simulink model "Q4_Sensor_Unpack"  (R2018b)
settings: Solver=VariableStepAuto  StartTime=0.0  StopTime=10.0  RelTol=1e-3
(part 2 of 2)

== matlab function Q4_Sensor_Unpack/message_unpack ==
  data: CAFDva_y_F_RadarData151 input; CAFDva_y_F_RadarData152 input; CAFDva_y_F_RadarData153 input; CAFDva_y_F_RadarData154 input; CAFDva_y_F_RadarData155 input; CAFDva_y_F_RadarData156 input; CAFDva_y_F_RadarData157 input; CAFDva_y_F_RadarData158 input; CAFDva_y_F_RadarData159 input; CAFDva_y_F_RadarData15A input; CAFDva_y_F_RadarData15B input; CAFDva_y_F_RadarData15C input; CAFDva_y_F_RadarData15D input; CAFDva_y_F_RadarData15E input; CAFDva_y_F_RadarData15F input; CAFDva_y_F_RadarData160 input; CAFDva_y_F_RadarData161 input; CAFDva_y_F_RadarData162 input; CAFDva_y_F_RadarData163 input; CAFDva_y_F_RadarData164 input; CAFDva_y_F_RadarData165 input; CAFDva_y_F_RadarData166 input; CAFDva_y_F_RadarData167 input; CAFDva_y_F_RadarData168 input; CAFDva_y_F_RadarData169 input; CAFDva_y_F_CameraData600 input; CAFDva_y_F_CameraData424 input; CAFDva_y_F_CameraData425 input; CAFDva_y_F_CameraData450 input; CAFDva_y_F_CameraData459 input; CAFDva_y_F_CameraData45A input; CAFDva_y_F_CameraData45B input; CAFDva_y_F_CameraData45C input; CAFDva_y_F_CameraData45D input; CAFDva_y_F_CameraData45E input; CAFDva_y_F_CameraData45F input; CAFDva_y_F_CameraData420 input; CAFDva_y_F_CameraData421 input; CAFDva_y_F_CameraData422 input; CAFDva_y_F_CameraData451 input; CAFDva_y_F_CameraData423 input; CAFDva_y_F_CameraData452 input; CAFDva_y_F_CameraData453 input; CAFDva_y_F_CameraData454 input; CAFDva_y_F_CameraData455 input; CAFDva_y_F_CameraData456 input; CAFDva_y_F_CameraData457 input; CAFDva_y_F_CameraData458 input; CAFDva_y_F_CameraData426 input; Radar_Timestamp output; Radar_status output; Radar_num output; Radar_P_long output; Radar_P_long_std output; Radar_P_latd output; Radar_P_latd_std output; Radar_P_Dis_cov output; Radar_Relative_V_long output; Radar_Relative_V_lat output; Radar_Relative_Acc_lat output; Radar_Relative_Acc_long output; Radar_Abs_V_long output; Radar_Abs_V_long_std output; Radar_Abs_V_long_acc output; Radar_Abs_V_long_acc_std output; Radar_Abs_V_lat output; Radar_Abs_V_lat_std output; Radar_Abs_V_lat_acc output; Radar_Abs_V_lat_acc_std output; Radar_Abs_V_cov output; Radar_Abs_V_acc_cov output; Radar_Class_type output; Radar_Class_prob output; Radar_Obj_length output; Radar_Obj_length_std output; Radar_Obj_width output; Radar_Obj_width_std output; Radar_Obj_height output; Radar_Obj_height_std output; Radar_Obj_id output; Radar_Obj_age output; Radar_Obj_referpoint output; Radar_Obj_Yaw output; Radar_Obj_Yaw_std output; Radar_Obj_Movementstatus output; Radar_Obj_Measurestatus output; Radar_Braking_allowed output; Radar_CrossSection output; Radar_Exist_prob output; IFC_obj_timestamp output; IFC_State output; IFC_ObjHdr_ObjCount output; IFC_VD_CIPV_ID output; FS_Out_Of_Calib output; FS_Rain output; FS_Fog output; FS_Splashes_0 output; FS_Sun_Ray_0 output; FS_Low_Sun_0 output; FS_Blur_Image_0 output; FS_Partial_Blockage_0 output; FS_Full_Blockage_0 output; FS_Frozen_Windshield_0 output; FS_Out_Of_Focus_0 output; IFC_obj_TTIPC_StdDev output; IFC_obj_abs_Ax output; IFC_obj_abs_Ay output; IFC_obj_Rel_Vx output; IFC_obj_Rel_Vy output; IFC_obj_Dx output; IFC_obj_Dy output; IFC_obj_abs_AxStdDev output; IFC_obj_abs_AyStdDev output; IFC_obj_Rel_VxStdDev output; IFC_obj_Rel_VyStdDev output; IFC_obj_DxStdDev output; IFC_obj_DyStdDev output; IFC_obj_Rel_VxValid output; IFC_obj_Rel_VyValid output; IFC_obj_Rel_VxStdDevValid output; IFC_obj_Rel_VyStdDevValid output; IFC_obj_ExistProb output; IFC_obj_TypeProb output; IFC_obj_Width output; IFC_obj_Height output; IFC_obj_LengthStdDev output; IFC_obj_WidthStdDev output; IFC_obj_HeightStdDev output; IFC_obj_PhiLeft output; IFC_obj_PhiRight output; IFC_obj_angle_3D output; IFC_obj_PhiLeftStdDev output; IFC_obj_PhiRightStdDev output; IFC_obj_angle_3DStdDev output; IFC_obj_angle_rate output; IFC_obj_angle_rate_StdDev output; IFC_obj_PhiBottom output; IFC_obj_PhiBottomStdDev output; IFC_obj_Measured output; IFC_obj_Heading output; IFC_obj_HeadingStdDev output; IFC_obj_HeadOrientation output; IFC_obj_Type output; IFC_obj_ID output; IFC_obj_TTIPC output; IFC_obj_DirIndicator output; IFC_obj_BrakeLight output; IFC_Line01_LineID output; IFC_Line01_ExistProb output; IFC_Line01_DxStart output; IFC_Line01_ColorClass output; IFC_Line01_DxEnd output; IFC_Line01_HeadingAngle output; IFC_Line01_Dy output; IFC_Line01_CurvChange output; IFC_Line01_Curv output; IFC_Line01_MeasureType output; IFC_Line01_LineWidth output; IFC_Line01_Type output; IFC_Line01_TypeConf output; IFC_Line02_LineID output; IFC_Line02_ExistProb output; IFC_Line02_DxStart output; IFC_Line02_ColorClass output; IFC_Line02_DxEnd output; IFC_Line02_HeadingAngle output; IFC_Line02_Dy output; IFC_Line02_CurvChange output; IFC_Line02_Curv output; IFC_Line02_MeasureType output; IFC_Line02_LineWidth output; IFC_Line02_Type output; IFC_Line02_TypeConf output; IFC_Line03_LineID output; IFC_Line03_ExistProb output; IFC_Line03_DxStart output; IFC_Line03_ColorClass output; IFC_Line03_DxEnd output; IFC_Line03_HeadingAngle output; IFC_Line03_Dy output; IFC_Line03_CurvChange output; IFC_Line03_Curv output; IFC_Line03_MeasureType output; IFC_Line03_LineWidth output; IFC_Line03_Type output; IFC_Line03_TypeConf output; IFC_Line04_LineID output; IFC_Line04_ExistProb output; IFC_Line04_DxStart output; IFC_Line04_ColorClass output; IFC_Line04_DxEnd output; IFC_Line04_HeadingAngle output; IFC_Line04_Dy output; IFC_Line04_CurvChange output; IFC_Line04_Curv output; IFC_Line04_MeasureType output; IFC_Line04_LineWidth output; IFC_Line04_Type output; IFC_Line04_TypeConf output; IFC_Roadedge01_LineID output; IFC_Roadedge01_ExistProb output; IFC_Roadedge01_DxStart output; IFC_Roadedge01_DxEnd output; IFC_Roadedge01_HeadingAngle output; IFC_Roadedge01_Dy output; IFC_Roadedge01_Curv output; IFC_Roadedge01_CurvChange output; IFC_Roadedge01_MeasureType output; IFC_Roadedge01_Type output; IFC_Roadedge02_LineID output; IFC_Roadedge02_ExistProb output; IFC_Roadedge02_DxStart output; IFC_Roadedge02_DxEnd output; IFC_Roadedge02_HeadingAngle output; IFC_Roadedge02_Dy output; IFC_Roadedge02_Curv output; IFC_Roadedge02_CurvChange output; IFC_Roadedge02_MeasureType output; IFC_Roadedge02_Type output; CAFDva_y_F_CameraData47E input
%% function for unpack and repack of canfd log data by liuyij 20210224
function [Radar_Timestamp,Radar_status,Radar_num,Radar_P_long,Radar_P_long_std,Radar_P_latd,Radar_P_latd_std,Radar_P_Dis_cov,...
    Radar_Relative_V_long,Radar_Relative_V_lat,Radar_Relative_Acc_lat,Radar_Relative_Acc_long,Radar_Abs_V_long,...
    Radar_Abs_V_long_std,Radar_Abs_V_long_acc,Radar_Abs_V_long_acc_std,Radar_Abs_V_lat,Radar_Abs_V_lat_std,Radar_Abs_V_lat_acc,...
    Radar_Abs_V_lat_acc_std,Radar_Abs_V_cov,Radar_Abs_V_acc_cov,Radar_Class_type,Radar_Class_prob,Radar_Obj_length,Radar_Obj_length_std,...
    Radar_Obj_width,Radar_Obj_width_std,Radar_Obj_height,Radar_Obj_height_std,Radar_Obj_id,Radar_Obj_age,Radar_Obj_referpoint,Radar_Obj_Yaw,...
    Radar_Obj_Yaw_std,Radar_Obj_Movementstatus,Radar_Obj_Measurestatus,Radar_Braking_allowed,Radar_CrossSection,Radar_Exist_prob,...
    IFC_obj_timestamp,IFC_State,IFC_ObjHdr_ObjCount,IFC_VD_CIPV_ID,...
    FS_Out_Of_Calib,FS_Rain,FS_Fog,FS_Splashes_0,FS_Sun_Ray_0,FS_Low_Sun_0,FS_Blur_Image_0,FS_Partial_Blockage_0,FS_Full_Blockage_0,FS_Frozen_Windshield_0,FS_Out_Of_Focus_0,...
    IFC_obj_TTIPC_StdDev,IFC_obj_abs_Ax,IFC_obj_abs_Ay,IFC_obj_Rel_Vx,IFC_obj_Rel_Vy,IFC_obj_Dx,IFC_obj_Dy,IFC_obj_abs_AxStdDev,IFC_obj_abs_AyStdDev,...
    IFC_obj_Rel_VxStdDev,IFC_obj_Rel_VyStdDev,IFC_obj_DxStdDev,IFC_obj_DyStdDev,IFC_obj_Rel_VxValid,IFC_obj_Rel_VyValid,IFC_obj_Rel_VxStdDevValid,...
    IFC_obj_Rel_VyStdDevValid,IFC_obj_ExistProb,IFC_obj_TypeProb,IFC_obj_Width,IFC_obj_Height,IFC_obj_LengthStdDev,IFC_obj_WidthStdDev,IFC_obj_HeightStdDev,...
    IFC_obj_PhiLeft,IFC_obj_PhiRight,IFC_obj_angle_3D,IFC_obj_PhiLeftStdDev,IFC_obj_PhiRightStdDev,IFC_obj_angle_3DStdDev,IFC_obj_angle_rate,...
    IFC_obj_angle_rate_StdDev,IFC_obj_PhiBottom,IFC_obj_PhiBottomStdDev,IFC_obj_Measured,IFC_obj_Heading,IFC_obj_HeadingStdDev,IFC_obj_HeadOrientation,...
    IFC_obj_Type,IFC_obj_ID,IFC_obj_TTIPC,IFC_obj_DirIndicator,IFC_obj_BrakeLight,...
    IFC_Line01_LineID,IFC_Line01_ExistProb,IFC_Line01_DxStart,IFC_Line01_ColorClass,IFC_Line01_DxEnd,IFC_Line01_HeadingAngle,IFC_Line01_Dy,...
    IFC_Line01_CurvChange,IFC_Line01_Curv,IFC_Line01_MeasureType,IFC_Line01_LineWidth,IFC_Line01_Type,IFC_Line01_TypeConf,...
    IFC_Line02_LineID,IFC_Line02_ExistProb,IFC_Line02_DxStart,IFC_Line02_ColorClass,IFC_Line02_DxEnd,IFC_Line02_HeadingAngle,IFC_Line02_Dy,...
    IFC_Line02_CurvChange,IFC_Line02_Curv,IFC_Line02_MeasureType,IFC_Line02_LineWidth,IFC_Line02_Type,IFC_Line02_TypeConf,...
    IFC_Line03_LineID,IFC_Line03_ExistProb,IFC_Line03_DxStart,IFC_Line03_ColorClass,IFC_Line03_DxEnd,IFC_Line03_HeadingAngle,IFC_Line03_Dy,...
    IFC_Line03_CurvChange,IFC_Line03_Curv,IFC_Line03_MeasureType,IFC_Line03_LineWidth,IFC_Line03_Type,IFC_Line03_TypeConf,...
    IFC_Line04_LineID,IFC_Line04_ExistProb,IFC_Line04_DxStart,IFC_Line04_ColorClass,IFC_Line04_DxEnd,IFC_Line04_HeadingAngle,IFC_Line04_Dy,...
    IFC_Line04_CurvChange,IFC_Line04_Curv,IFC_Line04_MeasureType,IFC_Line04_LineWidth,IFC_Line04_Type,IFC_Line04_TypeConf,...
    IFC_Roadedge01_LineID,IFC_Roadedge01_ExistProb,IFC_Roadedge01_DxStart,IFC_Roadedge01_DxEnd,IFC_Roadedge01_HeadingAngle,...
    IFC_Roadedge01_Dy,IFC_Roadedge01_Curv,IFC_Roadedge01_CurvChange,IFC_Roadedge01_MeasureType,IFC_Roadedge01_Type,...
    IFC_Roadedge02_LineID,IFC_Roadedge02_ExistProb,IFC_Roadedge02_DxStart,IFC_Roadedge02_DxEnd,IFC_Roadedge02_HeadingAngle,...
    IFC_Roadedge02_Dy,IFC_Roadedge02_Curv,IFC_Roadedge02_CurvChange,IFC_Roadedge02_MeasureType,IFC_Roadedge02_Type]...
    = sensor_unpack(CAFDva_y_F_RadarData151,CAFDva_y_F_RadarData152,CAFDva_y_F_RadarData153,CAFDva_y_F_RadarData154,...
    CAFDva_y_F_RadarData155,CAFDva_y_F_RadarData156,CAFDva_y_F_RadarData157,CAFDva_y_F_RadarData158,CAFDva_y_F_RadarData159,...
    CAFDva_y_F_RadarData15A,CAFDva_y_F_RadarData15B,CAFDva_y_F_RadarData15C,CAFDva_y_F_RadarData15D,CAFDva_y_F_RadarData15E,CAFDva_y_F_RadarData15F,...
    CAFDva_y_F_RadarData160,CAFDva_y_F_RadarData161,CAFDva_y_F_RadarData162,CAFDva_y_F_RadarData163,CAFDva_y_F_RadarData164,...
    CAFDva_y_F_RadarData165,CAFDva_y_F_RadarData166,CAFDva_y_F_RadarData167,CAFDva_y_F_RadarData168,CAFDva_y_F_RadarData169,...
    CAFDva_y_F_CameraData600,CAFDva_y_F_CameraData424,CAFDva_y_F_CameraData425,CAFDva_y_F_CameraData450,CAFDva_y_F_CameraData459,...
    CAFDva_y_F_CameraData45A,CAFDva_y_F_CameraData45B,CAFDva_y_F_CameraData45C,CAFDva_y_F_CameraData45D,CAFDva_y_F_CameraData45E,...
    CAFDva_y_F_CameraData45F,CAFDva_y_F_CameraData420,CAFDva_y_F_CameraData421,CAFDva_y_F_CameraData422,CAFDva_y_F_CameraData451,...
    CAFDva_y_F_CameraData423,CAFDva_y_F_CameraData452,CAFDva_y_F_CameraData453,CAFDva_y_F_CameraData454,CAFDva_y_F_CameraData455,...
    CAFDva_y_F_CameraData456,CAFDva_y_F_CameraData457,CAFDva_y_F_CameraData458,CAFDva_y_F_CameraData426,CAFDva_y_F_CameraData47E)

RADAR_MAX = uint8(24);
CAM_MAX = uint8(20);

%% output data initial 
% radar output
Radar_Timestamp = zeros(RADAR_MAX,1,'uint16');
Radar_status = uint8(0);
Radar_num = uint8(0);
Radar_P_long = zeros(RADAR_MAX,1,'single');
Radar_P_long_std= zeros(RADAR_MAX,1,'single');
Radar_P_latd= zeros(RADAR_MAX,1,'single');
Radar_P_latd_std= zeros(RADAR_MAX,1,'single');
Radar_P_Dis_cov= zeros(RADAR_MAX,1,'single');
Radar_Relative_V_long= zeros(RADAR_MAX,1,'single');
Radar_Relative_V_lat= zeros(RADAR_MAX,1,'single');
Radar_Relative_Acc_lat= zeros(RADAR_MAX,1,'single');
Radar_Relative_Acc_long= zeros(RADAR_MAX,1,'single');
Radar_Abs_V_long= zeros(RADAR_MAX,1,'single');
Radar_Abs_V_long_std= zeros(RADAR_MAX,1,'single');
Radar_Abs_V_long_acc= zeros(RADAR_MAX,1,'single');
Radar_Abs_V_long_acc_std= zeros(RADAR_MAX,1,'single');
Radar_Abs_V_lat= zeros(RADAR_MAX,1,'single');
Radar_Abs_V_lat_std= zeros(RADAR_MAX,1,'single');
Radar_Abs_V_lat_acc= zeros(RADAR_MAX,1,'single');
Radar_Abs_V_lat_acc_std= zeros(RADAR_MAX,1,'single');
Radar_Abs_V_cov= zeros(RADAR_MAX,1,'single');
Radar_Abs_V_acc_cov = zeros(RADAR_MAX,1,'single');
Radar_Class_type= zeros(RADAR_MAX,1,'uint8');
Radar_Class_prob= zeros(RADAR_MAX,1,'uint8');
Radar_Obj_length = zeros(RADAR_MAX,1,'single');
Radar_Obj_length_std = zeros(RADAR_MAX,1,'single');
Radar_Obj_width = zeros(RADAR_MAX,1,'single');
Radar_Obj_width_std = zeros(RADAR_MAX,1,'single');
Radar_Obj_height = zeros(RADAR_MAX,1,'single');
Radar_Obj_height_std = zeros(RADAR_MAX,1,'single');
Radar_Obj_id = zeros(RADAR_MAX,1,'uint8');
Radar_Obj_age = zeros(RADAR_MAX,1,'single');
Radar_Obj_referpoint = zeros(RADAR_MAX,1,'uint8');
Radar_Obj_Yaw = zeros(RADAR_MAX,1,'single');
Radar_Obj_Yaw_std = zeros(RADAR_MAX,1,'single');
Radar_Obj_Movementstatus = zeros(RADAR_MAX,1,'uint8');
Radar_Obj_Measurestatus = zeros(RADAR_MAX,1,'uint8');
Radar_Braking_allowed = zeros(RADAR_MAX,1,'uint8');
Radar_CrossSection = zeros(RADAR_MAX,1,'single');
Radar_Exist_prob = zeros(RADAR_MAX,1,'uint8');

% cam output
IFC_State = zeros(1,1,'uint8');
IFC_ObjHdr_ObjCount = zeros(1,1,'uint8');
IFC_VD_CIPV_ID = zeros(1,1,'uint8');

FS_Out_Of_Calib = zeros(1,1,'uint8');
FS_Rain = zeros(1,1,'uint8');
FS_Fog = zeros(1,1,'uint8');
FS_Splashes_0 = zeros(1,1,'uint8');
FS_Sun_Ray_0 = zeros(1,1,'uint8');
FS_Low_Sun_0 = zeros(1,1,'uint8');
FS_Blur_Image_0 = zeros(1,1,'uint8');
FS_Partial_Blockage_0 = zeros(1,1,'uint8');
FS_Full_Blockage_0 = zeros(1,1,'uint8');
FS_Frozen_Windshield_0 = zeros(1,1,'uint8');
FS_Out_Of_Focus_0 = zeros(1,1,'uint8');

IFC_obj_TTIPC_StdDev = zeros(CAM_MAX,1,'single');
IFC_obj_abs_Ax = zeros(CAM_MAX,1,'single');
IFC_obj_abs_Ay = zeros(CAM_MAX,1,'single');
IFC_obj_Rel_Vx = zeros(CAM_MAX,1,'single');
IFC_obj_Rel_Vy = zeros(CAM_MAX,1,'single');
IFC_obj_Dx = zeros(CAM_MAX,1,'single');
IFC_obj_Dy = zeros(CAM_MAX,1,'single');
IFC_obj_abs_AxStdDev = zeros(CAM_MAX,1,'single');
IFC_obj_abs_AyStdDev = zeros(CAM_MAX,1,'single');
IFC_obj_Rel_VxStdDev = zeros(CAM_MAX,1,'single');
IFC_obj_Rel_VyStdDev = zeros(CAM_MAX,1,'single');
IFC_obj_DxStdDev = zeros(CAM_MAX,1,'single');
IFC_obj_DyStdDev = zeros(CAM_MAX,1,'single');
IFC_obj_Rel_VxValid = zeros(CAM_MAX,1,'uint8');
IFC_obj_Rel_VyValid = zeros(CAM_MAX,1,'uint8');
IFC_obj_Rel_VxStdDevValid = zeros(CAM_MAX,1,'uint8');
IFC_obj_Rel_VyStdDevValid = zeros(CAM_MAX,1,'uint8');
IFC_obj_ExistProb = zeros(CAM_MAX,1,'single');
IFC_obj_TypeProb = zeros(CAM_MAX,1,'single');
IFC_obj_Width = zeros(CAM_MAX,1,'single');
IFC_obj_Height = zeros(CAM_MAX,1,'single');
IFC_obj_LengthStdDev = zeros(CAM_MAX,1,'single');
IFC_obj_WidthStdDev = zeros(CAM_MAX,1,'single');
IFC_obj_HeightStdDev = zeros(CAM_MAX,1,'single');
IFC_obj_PhiLeft = zeros(CAM_MAX,1,'single');
IFC_obj_PhiRight = zeros(CAM_MAX,1,'single');
IFC_obj_angle_3D = zeros(CAM_MAX,1,'single');
IFC_obj_PhiLeftStdDev = zeros(CAM_MAX,1,'single');
IFC_obj_PhiRightStdDev = zeros(CAM_MAX,1,'single');
IFC_obj_angle_3DStdDev = zeros(CAM_MAX,1,'single');
IFC_obj_angle_rate = zeros(CAM_MAX,1,'single');
IFC_obj_angle_rate_StdDev = zeros(CAM_MAX,1,'single');
IFC_obj_PhiBottom = zeros(CAM_MAX,1,'single');
IFC_obj_PhiBottomStdDev = zeros(CAM_MAX,1,'single');
IFC_obj_Measured = zeros(CAM_MAX,1,'uint8');
IFC_obj_Heading = zeros(CAM_MAX,1,'single');
IFC_obj_HeadingStdDev = zeros(CAM_MAX,1,'single');
IFC_obj_HeadOrientation = zeros(CAM_MAX,1,'uint8');
IFC_obj_Type = zeros(CAM_MAX,1,'uint8');
IFC_obj_ID = zeros(CAM_MAX,1,'uint8');
IFC_obj_TTIPC = zeros(CAM_MAX,1,'single');
IFC_obj_DirIndicator = zeros(CAM_MAX,1,'uint8');
IFC_obj_BrakeLight = zeros(CAM_MAX,1,'uint8');

IFC_obj_timestamp = zeros(CAM_MAX,1,'uint16');

IFC_Line01_LineID = zeros(1,1,'uint8');
IFC_Line01_ExistProb = zeros(1,1,'single');
IFC_Line01_DxStart = zeros(1,1,'single');
IFC_Line01_ColorClass = zeros(1,1,'uint8');
IFC_Line01_DxEnd = zeros(1,1,'single');
IFC_Line01_HeadingAngle = zeros(1,1,'single');
IFC_Line01_Dy = zeros(1,1,'single');
IFC_Line01_CurvChange = zeros(1,1,'single');
IFC_Line01_Curv = zeros(1,1,'single');
IFC_Line01_MeasureType = zeros(1,1,'uint8');
IFC_Line01_LineWidth = zeros(1,1,'single');
IFC_Line01_Type = zeros(1,1,'uint8');
IFC_Line01_TypeConf = zeros(1,1,'single');
IFC_Line02_LineID = zeros(1,1,'uint8');
IFC_Line02_ExistProb = zeros(1,1,'single');
IFC_Line02_DxStart = zeros(1,1,'single');
IFC_Line02_ColorClass = zeros(1,1,'uint8');
IFC_Line02_DxEnd = zeros(1,1,'single');
IFC_Line02_HeadingAngle = zeros(1,1,'single');
IFC_Line02_Dy = zeros(1,1,'single');
IFC_Line02_CurvChange = zeros(1,1,'single');
IFC_Line02_Curv = zeros(1,1,'single');
IFC_Line02_MeasureType = zeros(1,1,'uint8');
IFC_Line02_LineWidth = zeros(1,1,'single');
IFC_Line02_Type = zeros(1,1,'uint8');
IFC_Line02_TypeConf = zeros(1,1,'single');

IFC_Line03_LineID = zeros(1,1,'uint8');
IFC_Line03_ExistProb = zeros(1,1,'single');
IFC_Line03_DxStart = zeros(1,1,'single');
IFC_Line03_ColorClass = zeros(1,1,'uint8');
IFC_Line03_DxEnd = zeros(1,1,'single');
IFC_Line03_HeadingAngle = zeros(1,1,'single');
IFC_Line03_Dy = zeros(1,1,'single');
IFC_Line03_CurvChange = zeros(1,1,'single');
IFC_Line03_Curv = zeros(1,1,'single');
IFC_Line03_MeasureType = zeros(1,1,'uint8');
IFC_Line03_LineWidth = zeros(1,1,'single');
IFC_Line03_Type = zeros(1,1,'uint8');
IFC_Line03_TypeConf = zeros(1,1,'single');
IFC_Line04_LineID = zeros(1,1,'uint8');
IFC_Line04_ExistProb = zeros(1,1,'single');
IFC_Line04_DxStart = zeros(1,1,'single');
IFC_Line04_ColorClass = zeros(1,1,'uint8');
IFC_Line04_DxEnd = zeros(1,1,'single');
IFC_Line04_HeadingAngle = zeros(1,1,'single');
IFC_Line04_Dy = zeros(1,1,'single');
IFC_Line04_CurvChange = zeros(1,1,'single');
IFC_Line04_Curv = zeros(1,1,'single');
IFC_Line04_MeasureType = zeros(1,1,'uint8');
IFC_Line04_LineWidth = zeros(1,1,'single');
IFC_Line04_Type = zeros(1,1,'uint8');
IFC_Line04_TypeConf = zeros(1,1,'single');

IFC_Roadedge01_LineID = zeros(1,1,'uint8');
IFC_Roadedge01_ExistProb = zeros(1,1,'single');
IFC_Roadedge01_DxStart = zeros(1,1,'single');
IFC_Roadedge01_DxEnd = zeros(1,1,'single');
IFC_Roadedge01_HeadingAngle = zeros(1,1,'single');
IFC_Roadedge01_Dy = zeros(1,1,'single');
IFC_Roadedge01_Curv = zeros(1,1,'single');
IFC_Roadedge01_CurvChange = zeros(1,1,'single');
IFC_Roadedge01_MeasureType = zeros(1,1,'uint8');
IFC_Roadedge01_Type = zeros(1,1,'uint8');
IFC_Roadedge02_LineID = zeros(1,1,'uint8');
IFC_Roadedge02_ExistProb = zeros(1,1,'single');
IFC_Roadedge02_DxStart = zeros(1,1,'single');
IFC_Roadedge02_DxEnd = zeros(1,1,'single');
IFC_Roadedge02_HeadingAngle = zeros(1,1,'single');
IFC_Roadedge02_Dy = zeros(1,1,'single');
IFC_Roadedge02_Curv = zeros(1,1,'single');
IFC_Roadedge02_CurvChange = zeros(1,1,'single');
IFC_Roadedge02_MeasureType = zeros(1,1,'uint8');
IFC_Roadedge02_Type = zeros(1,1,'uint8');
%% put input message into temp matrix 
Radar_propty = zeros(66,RADAR_MAX,'uint8');
Cam_propty = zeros(66,CAM_MAX,'uint8');

%% get radar header property
[ Radar_status,Radar_num] = get_radar_header(CAFDva_y_F_RadarData151);

%% put radar canfd message into temp matrix 
Radar_propty = [CAFDva_y_F_RadarData152,CAFDva_y_F_RadarData153,CAFDva_y_F_RadarData154,CAFDva_y_F_RadarData155,...
    CAFDva_y_F_RadarData156,CAFDva_y_F_RadarData157,CAFDva_y_F_RadarData158,CAFDva_y_F_RadarData159,CAFDva_y_F_RadarData15A,...
    CAFDva_y_F_RadarData15B,CAFDva_y_F_RadarData15C,CAFDva_y_F_RadarData15D,CAFDva_y_F_RadarData15E,CAFDva_y_F_RadarData15F,...
    CAFDva_y_F_RadarData160,CAFDva_y_F_RadarData161,CAFDva_y_F_RadarData162,CAFDva_y_F_RadarData163,CAFDva_y_F_RadarData164,...
    CAFDva_y_F_RadarData165,CAFDva_y_F_RadarData166,CAFDva_y_F_RadarData167,CAFDva_y_F_RadarData168,CAFDva_y_F_RadarData169];
%% get radar obj property
[Radar_Timestamp,Radar_P_long,Radar_P_long_std,Radar_P_latd,Radar_P_latd_std,Radar_P_Dis_cov,...
    Radar_Relative_V_long,Radar_Relative_V_lat,Radar_Relative_Acc_lat,Radar_Relative_Acc_long,Radar_Abs_V_long,...
    Radar_Abs_V_long_std,Radar_Abs_V_long_acc,Radar_Abs_V_long_acc_std,Radar_Abs_V_lat,Radar_Abs_V_lat_std,Radar_Abs_V_lat_acc,...
    Radar_Abs_V_lat_acc_std,Radar_Abs_V_cov,Radar_Abs_V_acc_cov,Radar_Class_type,Radar_Class_prob,Radar_Obj_length,Radar_Obj_length_std,...
    Radar_Obj_width,Radar_Obj_width_std,Radar_Obj_height,Radar_Obj_height_std,Radar_Obj_id,Radar_Obj_age,Radar_Obj_referpoint,Radar_Obj_Yaw,...
    Radar_Obj_Yaw_std,Radar_Obj_Movementstatus,Radar_Obj_Measurestatus,Radar_Braking_allowed,Radar_CrossSection,Radar_Exist_prob]...
    = get_radar_obj_proty(Radar_propty,RADAR_MAX);

%% put cam canfd message into temp matrix 
Cam_propty =[CAFDva_y_F_CameraData450,CAFDva_y_F_CameraData451,CAFDva_y_F_CameraData452,CAFDva_y_F_CameraData453,...
    CAFDva_y_F_CameraData454,CAFDva_y_F_CameraData455,CAFDva_y_F_CameraData456,CAFDva_y_F_CameraData457,...
   CAFDva_y_F_CameraData458,CAFDva_y_F_CameraData459,CAFDva_y_F_CameraData45A,CAFDva_y_F_CameraData45B,...
    CAFDva_y_F_CameraData45C,CAFDva_y_F_CameraData45D,CAFDva_y_F_CameraData45E,CAFDva_y_F_CameraData45F,...
    CAFDva_y_F_CameraData420,CAFDva_y_F_CameraData421,CAFDva_y_F_CameraData422,CAFDva_y_F_CameraData423]; 
% %% get cam header property    
[IFC_State,IFC_ObjHdr_ObjCount,IFC_VD_CIPV_ID] = unpack_cam_status(CAFDva_y_F_CameraData426);
% %% get cam failsafe property
[FS_Out_Of_Calib,FS_Rain,FS_Fog,FS_Splashes_0,FS_Sun_Ray_0,FS_Low_Sun_0,FS_Blur_Image_0,FS_Partial_Blockage_0,...
    FS_Full_Blockage_0,FS_Frozen_Windshield_0,FS_Out_Of_Focus_0] = unpack_cam_failsafe(CAFDva_y_F_CameraData600);
%% get cam obj property
[IFC_obj_timestamp,IFC_obj_TTIPC_StdDev,IFC_obj_abs_Ax,IFC_obj_abs_Ay,IFC_obj_Rel_Vx,IFC_obj_Rel_Vy,IFC_obj_Dx,IFC_obj_Dy,...
    IFC_obj_abs_AxStdDev,IFC_obj_abs_AyStdDev,IFC_obj_Rel_VxStdDev,IFC_obj_Rel_VyStdDev,IFC_obj_DxStdDev,IFC_obj_DyStdDev,...
    IFC_obj_Rel_VxValid,IFC_obj_Rel_VyValid,IFC_obj_Rel_VxStdDevValid,IFC_obj_Rel_VyStdDevValid,IFC_obj_ExistProb,IFC_obj_TypeProb,...
    IFC_obj_Width,IFC_obj_Height,IFC_obj_LengthStdDev,IFC_obj_WidthStdDev,IFC_obj_HeightStdDev,IFC_obj_PhiLeft,IFC_obj_PhiRight,...
    IFC_obj_angle_3D,IFC_obj_PhiLeftStdDev,IFC_obj_PhiRightStdDev,IFC_obj_angle_3DStdDev,IFC_obj_angle_rate,IFC_obj_angle_rate_StdDev,...
    IFC_obj_PhiBottom,IFC_obj_PhiBottomStdDev,IFC_obj_Measured,IFC_obj_Heading,IFC_obj_HeadingStdDev,IFC_obj_HeadOrientation,IFC_obj_Type,...
    IFC_obj_ID,IFC_obj_TTIPC,IFC_obj_DirIndicator,IFC_obj_BrakeLight] = unpack_cam_obj_proty(Cam_propty,CAM_MAX);
%% get cam lane L0R0
[IFC_Line01_LineID,IFC_Line01_ExistProb,IFC_Line01_DxStart,IFC_Line01_ColorClass,IFC_Line01_DxEnd,IFC_Line01_HeadingAngle,IFC_Line01_Dy,...
    IFC_Line01_CurvChange,IFC_Line01_Curv,IFC_Line01_MeasureType,IFC_Line01_LineWidth,IFC_Line01_Type,IFC_Line01_TypeConf,...
    IFC_Line02_LineID,IFC_Line02_ExistProb,IFC_Line02_DxStart,IFC_Line02_ColorClass,IFC_Line02_DxEnd,IFC_Line02_HeadingAngle,IFC_Line02_Dy,...
    IFC_Line02_CurvChange,IFC_Line02_Curv,IFC_Line02_MeasureType,IFC_Line02_LineWidth,IFC_Line02_Type,IFC_Line02_TypeConf...
] = unpack_cam_L0R0(CAFDva_y_F_CameraData424);
%% get cam lane L1R1
[IFC_Line03_LineID,IFC_Line03_ExistProb,IFC_Line03_DxStart,IFC_Line03_ColorClass,IFC_Line03_DxEnd,IFC_Line03_HeadingAngle,IFC_Line03_Dy,...
    IFC_Line03_CurvChange,IFC_Line03_Curv,IFC_Line03_MeasureType,IFC_Line03_LineWidth,IFC_Line03_Type,IFC_Line03_TypeConf,...
    IFC_Line04_LineID,IFC_Line04_ExistProb,IFC_Line04_DxStart,IFC_Line04_ColorClass,IFC_Line04_DxEnd,IFC_Line04_HeadingAngle,IFC_Line04_Dy,...
    IFC_Line04_CurvChange,IFC_Line04_Curv,IFC_Line04_MeasureType,IFC_Line04_LineWidth,IFC_Line04_Type,IFC_Line04_TypeConf...
] = unpack_cam_L1R1(CAFDva_y_F_CameraData425);
%% get cam Roadedge
[IFC_Roadedge01_LineID,IFC_Roadedge01_ExistProb,IFC_Roadedge01_DxStart,IFC_Roadedge01_DxEnd,IFC_Roadedge01_HeadingAngle,...
    IFC_Roadedge01_Dy,IFC_Roadedge01_Curv,IFC_Roadedge01_CurvChange,IFC_Roadedge01_MeasureType,IFC_Roadedge01_Type,...
    IFC_Roadedge02_LineID,IFC_Roadedge02_ExistProb,IFC_Roadedge02_DxStart,IFC_Roadedge02_DxEnd,IFC_Roadedge02_HeadingAngle,...
    IFC_Roadedge02_Dy,IFC_Roadedge02_Curv,IFC_Roadedge02_CurvChange,IFC_Roadedge02_MeasureType,IFC_Roadedge02_Type...
] = unpack_cam_roadedge(CAFDva_y_F_CameraData47E);
end

function[radar_status,radar_obj_num]=get_radar_header(radar_header)
radar_status = bitshift(uint8(radar_header(6)),-5);
radar_obj_num = uint8(radar_header(12));
end

function[Radar_Timestamp,Radar_P_long,Radar_P_long_std,Radar_P_latd,Radar_P_latd_std,Radar_P_Dis_cov,...
    Radar_Relative_V_long,Radar_Relative_V_lat,Radar_Relative_Acc_lat,Radar_Relative_Acc_long,Radar_Abs_V_long,...
    Radar_Abs_V_long_std,Radar_Abs_V_long_acc,Radar_Abs_V_long_acc_std,Radar_Abs_V_lat,Radar_Abs_V_lat_std,Radar_Abs_V_lat_acc,...
    Radar_Abs_V_lat_acc_std,Radar_Abs_V_cov,Radar_Abs_V_acc_cov,Radar_Class_type,Radar_Class_prob,Radar_Obj_length,Radar_Obj_length_std,...
    Radar_Obj_width,Radar_Obj_width_std,Radar_Obj_height,Radar_Obj_height_std,Radar_Obj_id,Radar_Obj_age,Radar_Obj_referpoint,Radar_Obj_Yaw,...
    Radar_Obj_Yaw_std,Radar_Obj_Movementstatus,Radar_Obj_Measurestatus,Radar_Braking_allowed,Radar_CrossSection,Radar_Exist_prob]...
    =get_radar_obj_proty(radar_obj_data,RADAR_MAX)
Radar_Timestamp = zeros(RADAR_MAX,1,'uint16');
Radar_P_long = zeros(RADAR_MAX,1,'single');
Radar_P_long_std= zeros(RADAR_MAX,1,'single');
Radar_P_latd= zeros(RADAR_MAX,1,'single');
Radar_P_latd_std= zeros(RADAR_MAX,1,'single');
Radar_P_Dis_cov= zeros(RADAR_MAX,1,'single');
Radar_Relative_V_long= zeros(RADAR_MAX,1,'single');
Radar_Relative_V_lat= zeros(RADAR_MAX,1,'single');
Radar_Relative_Acc_lat= zeros(RADAR_MAX,1,'single');
Radar_Relative_Acc_long= zeros(RADAR_MAX,1,'single');
Radar_Abs_V_long= zeros(RADAR_MAX,1,'single');
Radar_Abs_V_long_std= zeros(RADAR_MAX,1,'single');
Radar_Abs_V_long_acc= zeros(RADAR_MAX,1,'single');
Radar_Abs_V_long_acc_std= zeros(RADAR_MAX,1,'single');
Radar_Abs_V_lat= zeros(RADAR_MAX,1,'single');
Radar_Abs_V_lat_std= zeros(RADAR_MAX,1,'single');
Radar_Abs_V_lat_acc= zeros(RADAR_MAX,1,'single');
Radar_Abs_V_lat_acc_std= zeros(RADAR_MAX,1,'single');
Radar_Abs_V_cov= zeros(RADAR_MAX,1,'single');
Radar_Abs_V_acc_cov = zeros(RADAR_MAX,1,'single');
Radar_Class_type= zeros(RADAR_MAX,1,'uint8');
Radar_Class_prob= zeros(RADAR_MAX,1,'uint8');
Radar_Obj_length = zeros(RADAR_MAX,1,'single');
Radar_Obj_length_std = zeros(RADAR_MAX,1,'single');
Radar_Obj_width = zeros(RADAR_MAX,1,'single');
Radar_Obj_width_std = zeros(RADAR_MAX,1,'single');
Radar_Obj_height = zeros(RADAR_MAX,1,'single');
Radar_Obj_height_std = zeros(RADAR_MAX,1,'single');
Radar_Obj_id = zeros(RADAR_MAX,1,'uint8');
Radar_Obj_age = zeros(RADAR_MAX,1,'single');
Radar_Obj_referpoint = zeros(RADAR_MAX,1,'uint8');
Radar_Obj_Yaw = zeros(RADAR_MAX,1,'single');
Radar_Obj_Yaw_std = zeros(RADAR_MAX,1,'single');
Radar_Obj_Movementstatus = zeros(RADAR_MAX,1,'uint8');
Radar_Obj_Measurestatus = zeros(RADAR_MAX,1,'uint8');
Radar_Braking_allowed = zeros(RADAR_MAX,1,'uint8');
Radar_CrossSection = zeros(RADAR_MAX,1,'single');
Radar_Exist_prob = zeros(RADAR_MAX,1,'uint8');
for i=1:RADAR_MAX   
    Radar_Timestamp(i) = bitor(bitshift(uint16(radar_obj_data(1,i)),8),uint16(radar_obj_data(2,i))); 
    Radar_P_long(i) =  single(fromBit_intel(48,13,radar_obj_data(3:52,i)))*single(0.05);
    Radar_P_long_std(i) = single(fromBit_intel(280,9,radar_obj_data(3:52,i)))*single(0.05);
    Radar_P_latd(i) = single(fromBit_intel(240,12,radar_obj_data(3:52,i)))*single(0.05)-single(100);
    Radar_P_latd_std(i) = single(fromBit_intel(256,9,radar_obj_data(3:52,i)))*single(0.05);
    Radar_P_Dis_cov(i) = single(fromBit_intel(224,10,radar_obj_data(3:52,i)))*single(0.05)-single(25);
    Radar_Relative_V_long(i) = single(fromBit_intel(344,12,radar_obj_data(3:52,i)))*single(0.05)-single(100);
    Radar_Relative_V_lat(i) = single(fromBit_intel(312,12,radar_obj_data(3:52,i)))*single(0.05)-single(100);
    Radar_Relative_Acc_lat(i) = single(fromBit_intel(296,10,radar_obj_data(3:52,i)))*single(0.05)-single(25);
    Radar_Relative_Acc_long(i) = single(fromBit_intel(328,10,radar_obj_data(3:52,i)))*single(0.05)-single(25);
    Radar_Abs_V_long(i) = single(fromBit_intel(192,12,radar_obj_data(3:52,i)))*single(0.05)-single(100);
    Radar_Abs_V_long_std(i) = single(fromBit_intel(128,9,radar_obj_data(3:52,i)))*single(0.02);
    Radar_Abs_V_long_acc(i) = single(fromBit_intel(176,10,radar_obj_data(3:52,i)))*single(0.05)-single(25);
    Radar_Abs_V_long_acc_std(i) = single(fromBit_intel(112,9,radar_obj_data(3:52,i)))*single(0.008);
    Radar_Abs_V_lat(i) = single(fromBit_intel(160,12,radar_obj_data(3:52,i)))*single(0.05)-single(100);
    Radar_Abs_V_lat_std(i) = single(fromBit_intel(96,9,radar_obj_data(3:52,i)))*single(0.02);
    Radar_Abs_V_lat_acc(i) = single(fromBit_intel(144,10,radar_obj_data(3:52,i)))*single(0.05)-single(25);
    Radar_Abs_V_lat_acc_std(i) = single(fromBit_intel(80,9,radar_obj_data(3:52,i)))*single(0.008);
    Radar_Abs_V_cov(i) = single(fromBit_intel(208,10,radar_obj_data(3:52,i)))*single(0.02)-single(8);
    Radar_Abs_V_acc_cov(i) = single(fromBit_intel(64,9,radar_obj_data(3:52,i)))*single(0.02)-single(5);
    Radar_Class_type(i) = uint8(fromBit_intel(10,3,radar_obj_data(3:52,i)));
    Radar_Class_prob(i) = uint8(fromBit_intel(73,7,radar_obj_data(3:52,i)));
    Radar_Obj_length(i) = single(fromBit_intel(272,8,radar_obj_data(3:52,i)))*single(0.1);
    Radar_Obj_length_std(i) = single(fromBit_intel(137,7,radar_obj_data(3:52,i)))*single(0.1);
    Radar_Obj_width(i) = single(fromBit_intel(186,6,radar_obj_data(3:52,i)))*single(0.1);
    Radar_Obj_width_std(i) = single(fromBit_intel(218,6,radar_obj_data(3:52,i)))*single(0.1);
    Radar_Obj_height(i) = single(fromBit_intel(105,6,radar_obj_data(3:52,i)))*single(0.1);
    Radar_Obj_height_std(i) = single(fromBit_intel(121,6,radar_obj_data(3:52,i)))*single(0.1);
    Radar_Obj_id(i) = uint8(fromBit_intel(0,8,radar_obj_data(3:52,i)));
    Radar_Obj_age(i) = single(fromBit_intel(16,15,radar_obj_data(3:52,i)))*single(0.01);
    Radar_Obj_referpoint(i) = uint8(fromBit_intel(40,4,radar_obj_data(3:52,i)));
    Radar_Obj_Yaw(i) = single(fromBit_intel(360,9,radar_obj_data(3:52,i)))*single(0.02)-single(3.142);
    Radar_Obj_Yaw_std(i) = single(fromBit_intel(376,9,radar_obj_data(3:52,i)))*single(0.02);
    Radar_Obj_Movementstatus(i) = uint8(fromBit_intel(13,3,radar_obj_data(3:52,i)));
    Radar_Obj_Measurestatus(i) = uint8(fromBit_intel(32,3,radar_obj_data(3:52,i)));
    Radar_Braking_allowed(i) = uint8(fromBit_intel(8,2,radar_obj_data(3:52,i)));
    Radar_CrossSection(i) = single(fromBit_intel(154,6,radar_obj_data(3:52,i)))*single(0.7)-single(20);
    Radar_Exist_prob(i) = uint8(fromBit_intel(89,7,radar_obj_data(3:52,i)));
end
end



%% intel format CANFD message unpack(without above timestamps)
function num  = fromBit_intel(startbit,length,all)
startbyte=floor(startbit/8)+1; %%get row of message lsb
endbit=rem(startbit,8);        %%get column of message lsb
byte1=bitshift(uint32(all(startbyte)),-endbit);%%rightshift lsb row
byte2=bitshift(uint32(all(startbyte+1)),8-endbit);%%leftshift msb row
byte3=bitshift(uint32(all(startbyte+2)),16-endbit);%%leftshift msb row
num=uint32(bitand(bitor(bitor(byte1,byte2),byte3),pow2(length)-uint32(1))); %%merge and pick valid bit of data
end

%% motorola format CANFD message unpack(without above timestamps)    
function num  = fromBit_motorola(startbit,length,all)
startbyte =uint8(floor(single(startbit)/single(8))+1);
endbit=uint8(rem(uint16(startbit),uint16(8)));
%%initial of byte3 and byte4
byte3 = uint32(0);
byte4 = uint32(0);
byte1=bitshift(uint32(all(startbyte)),-endbit);%右移
byte2=bitshift(uint32(all(startbyte-1)),8-endbit);%左移
if startbyte>uint8(3)
    byte3=bitshift(uint32(all(startbyte-2)),16-endbit);%左移
    byte4=bitshift(uint32(all(startbyte-3)),24-endbit);%左移
end
num=uint32(bitand(bitor(bitor(bitor(byte1,byte2),byte3),byte4),pow2(length)-uint32(1)));
end

function [IFC_obj_timestamp,IFC_obj_TTIPC_StdDev,IFC_obj_abs_Ax,IFC_obj_abs_Ay,IFC_obj_Rel_Vx,IFC_obj_Rel_Vy,IFC_obj_Dx,IFC_obj_Dy,IFC_obj_abs_AxStdDev,IFC_obj_abs_AyStdDev,IFC_obj_Rel_VxStdDev,IFC_obj_Rel_VyStdDev,IFC_obj_DxStdDev,IFC_obj_DyStdDev,IFC_obj_Rel_VxValid,IFC_obj_Rel_VyValid,IFC_obj_Rel_VxStdDevValid,IFC_obj_Rel_VyStdDevValid,IFC_obj_ExistProb,IFC_obj_TypeProb,IFC_obj_Width,IFC_obj_Height,IFC_obj_LengthStdDev,IFC_obj_WidthStdDev,IFC_obj_HeightStdDev,IFC_obj_PhiLeft,IFC_obj_PhiRight,IFC_obj_angle_3D,IFC_obj_PhiLeftStdDev,IFC_obj_PhiRightStdDev,IFC_obj_angle_3DStdDev,IFC_obj_angle_rate,IFC_obj_angle_rate_StdDev,IFC_obj_PhiBottom,IFC_obj_PhiBottomStdDev,IFC_obj_Measured,IFC_obj_Heading,IFC_obj_HeadingStdDev,IFC_obj_HeadOrientation,IFC_obj_Type,IFC_obj_ID,IFC_obj_TTIPC,IFC_obj_DirIndicator,IFC_obj_BrakeLight...
] = unpack_cam_obj_proty(Cam_obj,CAM_MAX)
IFC_obj_TTIPC_StdDev = zeros(CAM_MAX,1,'single');
IFC_obj_abs_Ax = zeros(CAM_MAX,1,'single');
IFC_obj_abs_Ay = zeros(CAM_MAX,1,'single');
IFC_obj_Rel_Vx = zeros(CAM_MAX,1,'single');
IFC_obj_Rel_Vy = zeros(CAM_MAX,1,'single');
IFC_obj_Dx = zeros(CAM_MAX,1,'single');
IFC_obj_Dy = zeros(CAM_MAX,1,'single');
IFC_obj_abs_AxStdDev = zeros(CAM_MAX,1,'single');
IFC_obj_abs_AyStdDev = zeros(CAM_MAX,1,'single');
IFC_obj_Rel_VxStdDev = zeros(CAM_MAX,1,'single');
IFC_obj_Rel_VyStdDev = zeros(CAM_MAX,1,'single');
IFC_obj_DxStdDev = zeros(CAM_MAX,1,'single');
IFC_obj_DyStdDev = zeros(CAM_MAX,1,'single');
IFC_obj_Rel_VxValid = zeros(CAM_MAX,1,'uint8');
IFC_obj_Rel_VyValid = zeros(CAM_MAX,1,'uint8');
IFC_obj_Rel_VxStdDevValid = zeros(CAM_MAX,1,'uint8');
IFC_obj_Rel_VyStdDevValid = zeros(CAM_MAX,1,'uint8');
IFC_obj_ExistProb = zeros(CAM_MAX,1,'single');
IFC_obj_TypeProb = zeros(CAM_MAX,1,'single');
IFC_obj_Width = zeros(CAM_MAX,1,'single');
IFC_obj_Height = zeros(CAM_MAX,1,'single');
IFC_obj_LengthStdDev = zeros(CAM_MAX,1,'single');
IFC_obj_WidthStdDev = zeros(CAM_MAX,1,'single');
IFC_obj_HeightStdDev = zeros(CAM_MAX,1,'single');
IFC_obj_PhiLeft = zeros(CAM_MAX,1,'single');
IFC_obj_PhiRight = zeros(CAM_MAX,1,'single');
IFC_obj_angle_3D = zeros(CAM_MAX,1,'single');
IFC_obj_PhiLeftStdDev = zeros(CAM_MAX,1,'single');
IFC_obj_PhiRightStdDev = zeros(CAM_MAX,1,'single');
IFC_obj_angle_3DStdDev = zeros(CAM_MAX,1,'single');
IFC_obj_angle_rate = zeros(CAM_MAX,1,'single');
IFC_obj_angle_rate_StdDev = zeros(CAM_MAX,1,'single');
IFC_obj_PhiBottom = zeros(CAM_MAX,1,'single');
IFC_obj_PhiBottomStdDev = zeros(CAM_MAX,1,'single');
IFC_obj_Measured = zeros(CAM_MAX,1,'uint8');
IFC_obj_Heading = zeros(CAM_MAX,1,'single');
IFC_obj_HeadingStdDev = zeros(CAM_MAX,1,'single');
IFC_obj_HeadOrientation = zeros(CAM_MAX,1,'uint8');
IFC_obj_Type = zeros(CAM_MAX,1,'uint8');
IFC_obj_ID = zeros(CAM_MAX,1,'uint8');
IFC_obj_TTIPC = zeros(CAM_MAX,1,'single');
IFC_obj_DirIndicator = zeros(CAM_MAX,1,'uint8');
IFC_obj_BrakeLight = zeros(CAM_MAX,1,'uint8');

IFC_obj_timestamp = zeros(CAM_MAX,1,'uint16');
for i=1:CAM_MAX
	IFC_obj_TTIPC_StdDev(i) = single(fromBit_intel(400,7,Cam_obj(3:56,i)))*single(0.0625)+single(0.0);
	IFC_obj_abs_Ax(i) = single(fromBit_intel(352,9,Cam_obj(3:56,i)))*single(0.05)+single(-10.3);
	IFC_obj_abs_Ay(i) = single(fromBit_intel(39,9,Cam_obj(3:56,i)))*single(0.05)+single(-10.3);
	IFC_obj_Rel_Vx(i) = single(fromBit_intel(76,13,Cam_obj(3:56,i)))*single(0.05)+single(-120.0);
	IFC_obj_Rel_Vy(i) = single(fromBit_intel(192,11,Cam_obj(3:56,i)))*single(0.05)+single(-50.0);
	IFC_obj_Dx(i) = single(fromBit_intel(50,14,Cam_obj(3:56,i)))*single(0.05)+single(-200.0);
	IFC_obj_Dy(i) = single(fromBit_intel(64,12,Cam_obj(3:56,i)))*single(0.05)+single(-100.0);
	IFC_obj_abs_AxStdDev(i) = single(fromBit_intel(24,8,Cam_obj(3:56,i)))*single(0.05)+single(0.0);
	IFC_obj_abs_AyStdDev(i) = single(fromBit_intel(216,8,Cam_obj(3:56,i)))*single(0.05)+single(0.0);
	IFC_obj_Rel_VxStdDev(i) = single(fromBit_intel(169,11,Cam_obj(3:56,i)))*single(0.05)+single(0.0);
	IFC_obj_Rel_VyStdDev(i) = single(fromBit_intel(96,10,Cam_obj(3:56,i)))*single(0.05)+single(0.0);
	IFC_obj_DxStdDev(i) = single(fromBit_intel(115,13,Cam_obj(3:56,i)))*single(0.05)+single(0.0);
	IFC_obj_DyStdDev(i) = single(fromBit_intel(128,11,Cam_obj(3:56,i)))*single(0.05)+single(0.0);
	IFC_obj_Rel_VxValid(i) = uint8(fromBit_intel(48,1,Cam_obj(3:56,i)));
	IFC_obj_Rel_VyValid(i) = uint8(fromBit_intel(49,1,Cam_obj(3:56,i)));
	IFC_obj_Rel_VxStdDevValid(i) = uint8(fromBit_intel(319,1,Cam_obj(3:56,i)));
	IFC_obj_Rel_VyStdDevValid(i) = uint8(fromBit_intel(351,1,Cam_obj(3:56,i)));
	IFC_obj_ExistProb(i) = single(fromBit_intel(89,7,Cam_obj(3:56,i)))*single(0.01)+single(0.0);
	IFC_obj_TypeProb(i) = single(fromBit_intel(32,7,Cam_obj(3:56,i)))*single(0.01)+single(0.0);
	IFC_obj_Width(i) = single(fromBit_intel(106,9,Cam_obj(3:56,i)))*single(0.01)+single(0.4);
	IFC_obj_Height(i) = single(fromBit_intel(288,9,Cam_obj(3:56,i)))*single(0.01)+single(0.0);
	IFC_obj_LengthStdDev(i) = single(fromBit_intel(344,7,Cam_obj(3:56,i)))*single(0.05)+single(0.0);
	IFC_obj_WidthStdDev(i) = single(fromBit_intel(385,7,Cam_obj(3:56,i)))*single(0.01)+single(0.0);
	IFC_obj_HeightStdDev(i) = single(fromBit_intel(297,7,Cam_obj(3:56,i)))*single(0.01)+single(0.0);
	IFC_obj_PhiLeft(i) = single(fromBit_intel(256,14,Cam_obj(3:56,i)))*single(0.0002)+single(-1.571);
	IFC_obj_PhiRight(i) = single(fromBit_intel(270,14,Cam_obj(3:56,i)))*single(0.0002)+single(-1.571);
	IFC_obj_angle_3D(i) = single(fromBit_intel(237,14,Cam_obj(3:56,i)))*single(0.0002)+single(-1.571);
	IFC_obj_PhiLeftStdDev(i) = single(fromBit_intel(224,13,Cam_obj(3:56,i)))*single(0.0002)+single(0.0);
	IFC_obj_PhiRightStdDev(i) = single(fromBit_intel(139,13,Cam_obj(3:56,i)))*single(0.0002)+single(0.0);
	IFC_obj_angle_3DStdDev(i) = single(fromBit_intel(203,13,Cam_obj(3:56,i)))*single(0.0002)+single(0.0);
	IFC_obj_angle_rate(i) = single(fromBit_intel(180,12,Cam_obj(3:56,i)))*single(0.002)+single(-2.234);
	IFC_obj_angle_rate_StdDev(i) = single(fromBit_intel(370,11,Cam_obj(3:56,i)))*single(0.002)+single(0.0);
	IFC_obj_PhiBottom(i) = single(fromBit_intel(330,14,Cam_obj(3:56,i)))*single(0.0002)+single(-1.571);
	IFC_obj_PhiBottomStdDev(i) = single(fromBit_intel(304,13,Cam_obj(3:56,i)))*single(0.0002)+single(0.0);
	IFC_obj_Measured(i) = uint8(fromBit_intel(317,2,Cam_obj(3:56,i)));
	IFC_obj_Heading(i) = single(fromBit_intel(320,10,Cam_obj(3:56,i)))*single(0.01)+single(-3.14);
	IFC_obj_HeadingStdDev(i) = single(fromBit_intel(361,9,Cam_obj(3:56,i)))*single(0.01)+single(0.0);
	IFC_obj_HeadOrientation(i) = uint8(fromBit_intel(284,4,Cam_obj(3:56,i)));
	IFC_obj_Type(i) = uint8(fromBit_intel(381,3,Cam_obj(3:56,i)));
	IFC_obj_ID(i) = uint8(fromBit_intel(392,8,Cam_obj(3:56,i)));
	IFC_obj_TTIPC(i) = single(fromBit_intel(408,11,Cam_obj(3:56,i)))*single(0.01)+single(-8.0);
	IFC_obj_DirIndicator(i) = uint8(fromBit_intel(253,3,Cam_obj(3:56,i)));
	IFC_obj_BrakeLight(i) = uint8(fromBit_intel(384,1,Cam_obj(3:56,i)));
	IFC_obj_timestamp(i) =  bitor(bitshift(uint16(Cam_obj(1,i)),8),uint16(Cam_obj(2,i)));
end
end

function [IFC_State,IFC_ObjHdr_ObjCount,IFC_VD_CIPV_ID...
] = unpack_cam_status(IFC_Status)

IFC_State = uint8(fromBit_intel(32,4,IFC_Status(3:11)));
IFC_ObjHdr_ObjCount = uint8(fromBit_intel(24,7,IFC_Status(3:11)));
IFC_VD_CIPV_ID = uint8(fromBit_intel(48,8,IFC_Status(3:11)));
end

function [FS_Out_Of_Calib,FS_Rain,FS_Fog,FS_Splashes_0,FS_Sun_Ray_0,FS_Low_Sun_0,FS_Blur_Image_0,FS_Partial_Blockage_0,FS_Full_Blockage_0,FS_Frozen_Windshield_0,FS_Out_Of_Focus_0...
] = unpack_cam_failsafe(IFC_Failsafe)

FS_Out_Of_Calib = uint8(fromBit_intel(30,3,IFC_Failsafe(3:8)));
FS_Rain = uint8(fromBit_intel(24,3,IFC_Failsafe(3:8)));
FS_Fog = uint8(fromBit_intel(21,3,IFC_Failsafe(3:8)));
FS_Splashes_0 = uint8(fromBit_intel(15,3,IFC_Failsafe(3:8)));
FS_Sun_Ray_0 = uint8(fromBit_intel(18,3,IFC_Failsafe(3:8)));
FS_Low_Sun_0 = uint8(fromBit_intel(12,3,IFC_Failsafe(3:8)));
FS_Blur_Image_0 = uint8(fromBit_intel(9,3,IFC_Failsafe(3:8)));
FS_Partial_Blockage_0 = uint8(fromBit_intel(27,3,IFC_Failsafe(3:8)));
FS_Full_Blockage_0 = uint8(fromBit_intel(6,3,IFC_Failsafe(3:8)));
FS_Frozen_Windshield_0 = uint8(fromBit_intel(3,3,IFC_Failsafe(3:8)));
FS_Out_Of_Focus_0 = uint8(fromBit_intel(0,3,IFC_Failsafe(3:8)));
end

function [IFC_Line01_LineID,IFC_Line01_ExistProb,IFC_Line01_DxStart,IFC_Line01_ColorClass,IFC_Line01_DxEnd,IFC_Line01_HeadingAngle,IFC_Line01_Dy,IFC_Line01_CurvChange,IFC_Line01_Curv,IFC_Line01_MeasureType,IFC_Line01_LineWidth,IFC_Line01_Type,IFC_Line01_TypeConf,IFC_Line02_LineID,IFC_Line02_ExistProb,IFC_Line02_DxStart,IFC_Line02_ColorClass,IFC_Line02_DxEnd,IFC_Line02_HeadingAngle,IFC_Line02_Dy,IFC_Line02_CurvChange,IFC_Line02_Curv,IFC_Line02_MeasureType,IFC_Line02_LineWidth,IFC_Line02_Type,IFC_Line02_TypeConf...
] = unpack_cam_L0R0(IFC_L0_R0)

IFC_Line01_LineID = uint8(fromBit_intel(24,8,IFC_L0_R0(3:40)));
IFC_Line01_ExistProb = single(fromBit_intel(272,6,IFC_L0_R0(3:40)))*single(0.02)+single(0.0);
IFC_Line01_DxStart = single(fromBit_intel(128,15,IFC_L0_R0(3:40)))*single(0.01)+single(0.0);
IFC_Line01_ColorClass = uint8(fromBit_intel(84,3,IFC_L0_R0(3:40)));
IFC_Line01_DxEnd = single(fromBit_intel(32,15,IFC_L0_R0(3:40)))*single(0.01)+single(0.0);
IFC_Line01_HeadingAngle = single(fromBit_intel(111,9,IFC_L0_R0(3:40)))*single(0.01)+single(-2.0);
IFC_Line01_Dy = single(fromBit_intel(47,13,IFC_L0_R0(3:40)))*single(0.01)+single(-30.0);
IFC_Line01_CurvChange = single(fromBit_intel(64,20,IFC_L0_R0(3:40)))*single(5e-08)+single(-0.024);
IFC_Line01_Curv = single(fromBit_intel(96,15,IFC_L0_R0(3:40)))*single(1.6e-05)+single(-0.25);
IFC_Line01_MeasureType = uint8(fromBit_intel(180,2,IFC_L0_R0(3:40)));
IFC_Line01_LineWidth = single(fromBit_intel(120,7,IFC_L0_R0(3:40)))*single(0.01)+single(0.0);
IFC_Line01_Type = uint8(fromBit_intel(60,4,IFC_L0_R0(3:40)));
IFC_Line01_TypeConf = single(fromBit_intel(223,7,IFC_L0_R0(3:40)))*single(0.01)+single(0.0);
IFC_Line02_LineID = uint8(fromBit_intel(184,8,IFC_L0_R0(3:40)));
IFC_Line02_ExistProb = single(fromBit_intel(259,6,IFC_L0_R0(3:40)))*single(0.02)+single(0.0);
IFC_Line02_DxStart = single(fromBit_intel(192,15,IFC_L0_R0(3:40)))*single(0.01)+single(0.0);
IFC_Line02_ColorClass = uint8(fromBit_intel(220,3,IFC_L0_R0(3:40)));
IFC_Line02_DxEnd = single(fromBit_intel(143,15,IFC_L0_R0(3:40)))*single(0.01)+single(0.0);
IFC_Line02_HeadingAngle = single(fromBit_intel(230,9,IFC_L0_R0(3:40)))*single(0.01)+single(-2.0);
IFC_Line02_Dy = single(fromBit_intel(207,13,IFC_L0_R0(3:40)))*single(0.01)+single(-30.0);
IFC_Line02_CurvChange = single(fromBit_intel(160,20,IFC_L0_R0(3:40)))*single(5e-08)+single(-0.024);
IFC_Line02_Curv = single(fromBit_intel(240,15,IFC_L0_R0(3:40)))*single(1.6e-05)+single(-0.25);
IFC_Line02_MeasureType = uint8(fromBit_intel(278,2,IFC_L0_R0(3:40)));
IFC_Line02_LineWidth = single(fromBit_intel(265,7,IFC_L0_R0(3:40)))*single(0.01)+single(0.0);
IFC_Line02_Type = uint8(fromBit_intel(255,4,IFC_L0_R0(3:40)));
IFC_Line02_TypeConf = single(fromBit_intel(280,7,IFC_L0_R0(3:40)))*single(0.01)+single(0.0);
end

function [IFC_Line03_LineID,IFC_Line03_ExistProb,IFC_Line03_DxStart,IFC_Line03_ColorClass,IFC_Line03_DxEnd,IFC_Line03_HeadingAngle,IFC_Line03_Dy,IFC_Line03_CurvChange,IFC_Line03_Curv,IFC_Line03_MeasureType,IFC_Line03_LineWidth,IFC_Line03_Type,IFC_Line03_TypeConf,IFC_Line04_LineID,IFC_Line04_ExistProb,IFC_Line04_DxStart,IFC_Line04_ColorClass,IFC_Line04_DxEnd,IFC_Line04_HeadingAngle,IFC_Line04_Dy,IFC_Line04_CurvChange,IFC_Line04_Curv,IFC_Line04_MeasureType,IFC_Line04_LineWidth,IFC_Line04_Type,IFC_Line04_TypeConf...
] = unpack_cam_L1R1(IFC_L1_R1)

IFC_Line03_LineID = uint8(fromBit_intel(24,8,IFC_L1_R1(3:40)));
IFC_Line03_ExistProb = single(fromBit_intel(272,6,IFC_L1_R1(3:40)))*single(0.02)+single(0.0);
IFC_Line03_DxStart = single(fromBit_intel(128,15,IFC_L1_R1(3:40)))*single(0.01)+single(0.0);
IFC_Line03_ColorClass = uint8(fromBit_intel(84,3,IFC_L1_R1(3:40)));
IFC_Line03_DxEnd = single(fromBit_intel(32,15,IFC_L1_R1(3:40)))*single(0.01)+single(0.0);
IFC_Line03_HeadingAngle = single(fromBit_intel(111,9,IFC_L1_R1(3:40)))*single(0.01)+single(-2.0);
IFC_Line03_Dy = single(fromBit_intel(47,13,IFC_L1_R1(3:40)))*single(0.01)+single(-30.0);
IFC_Line03_CurvChange = single(fromBit_intel(64,20,IFC_L1_R1(3:40)))*single(5e-08)+single(-0.024);
IFC_Line03_Curv = single(fromBit_intel(96,15,IFC_L1_R1(3:40)))*single(1.6e-05)+single(-0.25);
IFC_Line03_MeasureType = uint8(fromBit_intel(180,2,IFC_L1_R1(3:40)));
IFC_Line03_LineWidth = single(fromBit_intel(120,7,IFC_L1_R1(3:40)))*single(0.01)+single(0.0);
IFC_Line03_Type = uint8(fromBit_intel(60,4,IFC_L1_R1(3:40)));
IFC_Line03_TypeConf = single(fromBit_intel(223,7,IFC_L1_R1(3:40)))*single(0.01)+single(0.0);
IFC_Line04_LineID = uint8(fromBit_intel(184,8,IFC_L1_R1(3:40)));
IFC_Line04_ExistProb = single(fromBit_intel(259,6,IFC_L1_R1(3:40)))*single(0.02)+single(0.0);
IFC_Line04_DxStart = single(fromBit_intel(192,15,IFC_L1_R1(3:40)))*single(0.01)+single(0.0);
IFC_Line04_ColorClass = uint8(fromBit_intel(220,3,IFC_L1_R1(3:40)));
IFC_Line04_DxEnd = single(fromBit_intel(143,15,IFC_L1_R1(3:40)))*single(0.01)+single(0.0);
IFC_Line04_HeadingAngle = single(fromBit_intel(230,9,IFC_L1_R1(3:40)))*single(0.01)+single(-2.0);
IFC_Line04_Dy = single(fromBit_intel(207,13,IFC_L1_R1(3:40)))*single(0.01)+single(-30.0);
IFC_Line04_CurvChange = single(fromBit_intel(160,20,IFC_L1_R1(3:40)))*single(5e-08)+single(-0.024);
IFC_Line04_Curv = single(fromBit_intel(240,15,IFC_L1_R1(3:40)))*single(1.6e-05)+single(-0.25);
IFC_Line04_MeasureType = uint8(fromBit_intel(278,2,IFC_L1_R1(3:40)));
IFC_Line04_LineWidth = single(fromBit_intel(265,7,IFC_L1_R1(3:40)))*single(0.01)+single(0.0);
IFC_Line04_Type = uint8(fromBit_intel(255,4,IFC_L1_R1(3:40)));
IFC_Line04_TypeConf = single(fromBit_intel(280,7,IFC_L1_R1(3:40)))*single(0.01)+single(0.0);
end

function [IFC_Roadedge01_LineID,IFC_Roadedge01_ExistProb,IFC_Roadedge01_DxStart,IFC_Roadedge01_DxEnd,IFC_Roadedge01_HeadingAngle,IFC_Roadedge01_Dy,IFC_Roadedge01_Curv,IFC_Roadedge01_CurvChange,IFC_Roadedge01_MeasureType,IFC_Roadedge01_Type,IFC_Roadedge02_LineID,IFC_Roadedge02_ExistProb,IFC_Roadedge02_DxStart,IFC_Roadedge02_DxEnd,IFC_Roadedge02_HeadingAngle,IFC_Roadedge02_Dy,IFC_Roadedge02_Curv,IFC_Roadedge02_CurvChange,IFC_Roadedge02_MeasureType,IFC_Roadedge02_Type...
] = unpack_cam_roadedge(IFC_Roadedge)

IFC_Roadedge01_LineID = uint8(fromBit_intel(0,8,IFC_Roadedge(3:32)));
IFC_Roadedge01_ExistProb = single(fromBit_intel(8,6,IFC_Roadedge(3:32)))*single(0.02)+single(0.0);
IFC_Roadedge01_DxStart = single(fromBit_intel(14,15,IFC_Roadedge(3:32)))*single(0.01)+single(0.0);
IFC_Roadedge01_DxEnd = single(fromBit_intel(64,15,IFC_Roadedge(3:32)))*single(0.01)+single(0.0);
IFC_Roadedge01_HeadingAngle = single(fromBit_intel(181,9,IFC_Roadedge(3:32)))*single(0.01)+single(-2.0);
IFC_Roadedge01_Dy = single(fromBit_intel(219,13,IFC_Roadedge(3:32)))*single(0.01)+single(-30.0);
IFC_Roadedge01_Curv = single(fromBit_intel(79,15,IFC_Roadedge(3:32)))*single(1.6e-05)+single(-0.25);
IFC_Roadedge01_CurvChange = single(fromBit_intel(32,20,IFC_Roadedge(3:32)))*single(5e-08)+single(-0.024);
IFC_Roadedge01_MeasureType = uint8(fromBit_intel(29,2,IFC_Roadedge(3:32)));
IFC_Roadedge01_Type = uint8(fromBit_intel(192,4,IFC_Roadedge(3:32)));
IFC_Roadedge02_LineID = uint8(fromBit_intel(56,8,IFC_Roadedge(3:32)));
IFC_Roadedge02_ExistProb = single(fromBit_intel(162,6,IFC_Roadedge(3:32)))*single(0.02)+single(0.0);
IFC_Roadedge02_DxStart = single(fromBit_intel(97,15,IFC_Roadedge(3:32)))*single(0.01)+single(0.0);
IFC_Roadedge02_DxEnd = single(fromBit_intel(112,15,IFC_Roadedge(3:32)))*single(0.01)+single(0.0);
IFC_Roadedge02_HeadingAngle = single(fromBit_intel(143,9,IFC_Roadedge(3:32)))*single(0.01)+single(-2.0);
IFC_Roadedge02_Dy = single(fromBit_intel(168,13,IFC_Roadedge(3:32)))*single(0.01)+single(-30.0);
IFC_Roadedge02_Curv = single(fromBit_intel(128,15,IFC_Roadedge(3:32)))*single(1.6e-05)+single(-0.25);
IFC_Roadedge02_CurvChange = single(fromBit_intel(196,20,IFC_Roadedge(3:32)))*single(5e-08)+single(-0.024);
IFC_Roadedge02_MeasureType = uint8(fromBit_intel(94,2,IFC_Roadedge(3:32)));
IFC_Roadedge02_Type = uint8(fromBit_intel(52,4,IFC_Roadedge(3:32)));
end
